simulink model "mmc"  (R2025a)
settings: Solver=VariableStepAuto  StartTime=0.0  StopTime=10  RelTol=1e-3
libraries: nesl_utility x145, ee_lib x103, fl_lib x100
(part 1 of 13)
settings Model: Creator=tanus  LastModifiedBy=tanus

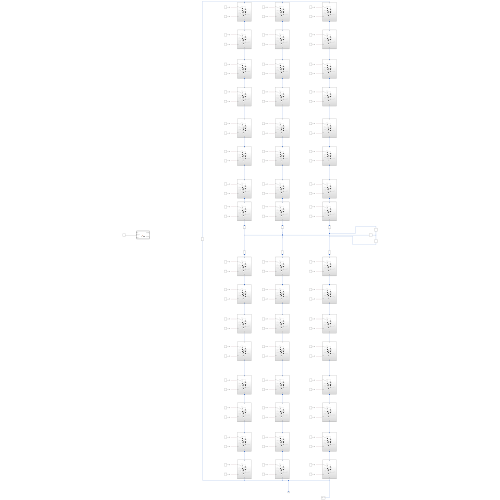
[thumbnail: Simulink's stored preview of the top-level diagram]
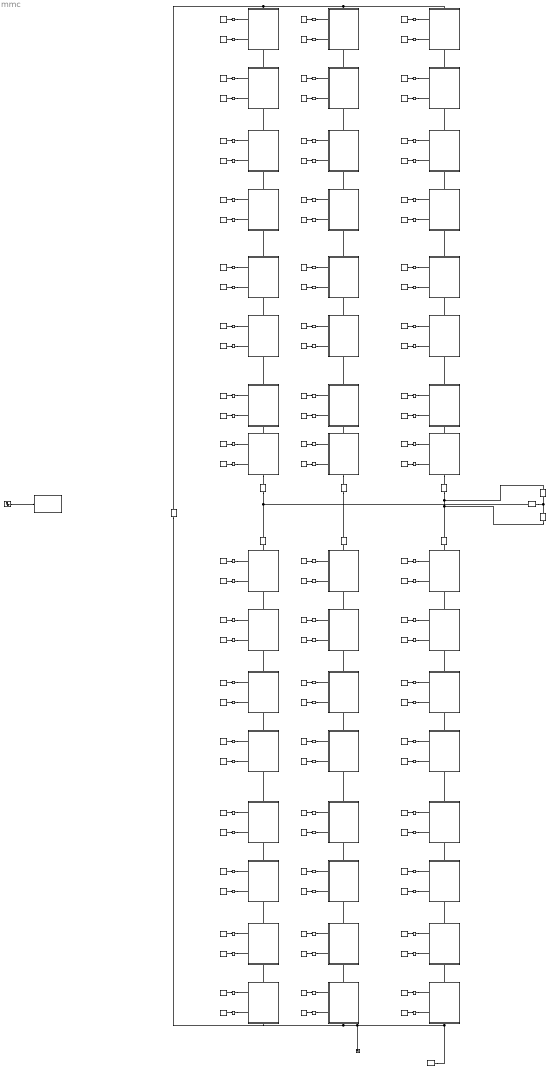
== system mmc ==
  Constant{1..96} (96 alike) : Constant  Value=10
  Electrical Reference : fl_lib/Electrical/Electrical Elements/Electrical Reference
  Inductor{6..11} (6 alike) : ee_lib/Passive/Inductor  l=1e-3 H  enable_L_tol=ee.enum.toleranceApplication.none  L_tol=20  tol_distribution=ee.enum.toleranceDistribution.uniform  nSigma=4  r=0 Ohm  g=1e-9 1/Ohm  enable_operating_limits=ee.enum.enable.no  operating_limit_action=ee.enum.passive.reportOpLim.warn  max_working_current=1 A  power_rating=1 W  i_L_specify=off  i_L_priority=High  i_L=0 A  i_L_nominal_specify=off  i_L_nominal_value=1  i_L_nominal_unit=A
  MATLAB Function : MATLAB Function  TreatAsAtomicUnit=on
  Resistor : fl_lib/Electrical/Electrical Elements/Resistor  R=1 Ohm  i_specify=off  i_priority=None  i=0 A  i_nominal_specify=off  i_nominal_value=1  i_nominal_unit=A  v_specify=off  v_priority=None  v=0 V  v_nominal_specify=off  v_nominal_value=1  v_nominal_unit=V
  Resistor1 : fl_lib/Electrical/Electrical Elements/Resistor  R=1 Ohm  i_specify=off  i_priority=None  i=0 A  i_nominal_specify=off  i_nominal_value=1  i_nominal_unit=A  v_specify=off  v_priority=None  v=0 V  v_nominal_specify=off  v_nominal_value=1  v_nominal_unit=V
  Resistor2 : fl_lib/Electrical/Electrical Elements/Resistor  R=1 Ohm  i_specify=off  i_priority=None  i=0 A  i_nominal_specify=off  i_nominal_value=1  i_nominal_unit=A  v_specify=off  v_priority=None  v=0 V  v_nominal_specify=off  v_nominal_value=1  v_nominal_unit=V
  Simulink-PS Converter{1..96} (96 alike) : nesl_utility/Simulink-PS Converter  PhysicalDomain=network_engine_domain  SubClassName=ps_input  LeftPortType=input  RightPortType=output  PseudoPeriodic=off  Frequencies=[]  NoiseDistribution=none  NoiseParameters=[]  Unit=1  AffineConversion=off  FilteringAndDerivatives=provide  SimscapeFilterOrder=1  InputFilterTimeConstant=0.001  UdotUserProvided=0
  Sine Wave : Sin  SampleTime=0
  Solver Configuration1 : nesl_utility/Solver Configuration  PhysicalDomain=network_engine_domain  SubClassName=solver  LeftPortType=input  RightPortType=generic  Tones=[]  Harmonics=[]  SimulateNoise=off  Profile=off  UseLocalSampling=off  EnableSwitchedLinearOptims=on  FrequencyDomain=off  UseCCode=off  RelTol=0.001  AbsTol=0.001  MinStep=1e-09  ToWorkspace=off  RevertToSquareIcSolve=off  NumHomotopyIterations=100  PhasorMode=off  PhasorModeNumHarmonics=1  ConsistencySolver=NEWTON_XTOL_AFTER_FTOL  IndexReductionMethod=DerivativeReplacement  DoDC=off  ResidualTolerance=1e-09  ConsistencyTolSource=GLOBAL  ConsistencyAbsTol=0.001  ConsistencyRelTol=0.001  ConsistencyTolFactor=0.001  UseLocalSolver=off  LocalSolverChoice=NE_BACKWARD_EULER_ADVANCER  ResolveIndetEquations=on  FunctionEvalNumThread=1  LocalSolverSampleTime=0.001  DoFixedCost=off  MaxNonlinIter=3  MaxModeIter=2  ComputeImpulses=off  ImpulseIterations=2  LinearAlgebra=auto  LinearAlgebraNumThread=0  EquationFormulation=NE_TIME_EF  DelaysMemoryBudget=1024  AutomaticFiltering=on  FilteringTimeConstant=0.001  PartitionStorageMethod=AS_NEEDED  PartitionMemoryBudget=1024  PartitionMethod=ROBUST  MultibodyUseLocalSolver=off  MultibodyLocalSolverChoice=ODE1  MultibodyLocalSolverSampleTime=0.001
  Subsystem1 : Subsystem
      settings: PortSchema="{\"entries\":[{\"content\":{\"sides\":[{\"content\":{\"connectorIds\":[\"LConn1\",\"LConn2\"]},\"type\":\"ConnectorPlacement.EquallySpacedRectSide\",\"uuid\":\"15b6a701-c482-4ab4-b894-e969b74b8fe7\"},{\"content\":{\"side\":\"RIGHT\"},\"type\":\"ConnectorPlacement.EquallySpacedRectSide\",\"uuid\":\"d0e695dd-06b6-4831-9b12-69abc92aa4b4\"},{\"content\":{\"connectorIds\":[\"LConn3\"],\"side\":\"TOP\"},\"type\":\"ConnectorPlacement.EquallySpacedRectSide\",\"uuid\":\"2d8cca64-5216-4108-8582-3d735b4d6af0\"},{\"content\":{\"connectorIds\":[\"RConn1\"],\"side\":\"BOTTOM\"},\"type\":\"ConnectorPlacement.EquallySpacedRectSide\",\"uuid\":\"da22ed5b-3a7b-44e1-acef-3ebda742cad5\"}]},\"type\":\"ConnectorPlacement.EquallySpacedConnector\",\"uuid\":\"49f96526-0040-486f-9e93-d2a8b3aa1224\"}],\"packageUris\":[\"http://schema.mathworks.com/mf0/Connector/R2020b\"],\"version\":\"1.0\"}"
  Subsystem10 : Subsystem
      settings: PortSchema="{\"entries\":[{\"content\":{\"sides\":[{\"content\":{\"connectorIds\":[\"LConn1\",\"LConn2\"]},\"type\":\"ConnectorPlacement.EquallySpacedRectSide\",\"uuid\":\"15b6a701-c482-4ab4-b894-e969b74b8fe7\"},{\"content\":{\"side\":\"RIGHT\"},\"type\":\"ConnectorPlacement.EquallySpacedRectSide\",\"uuid\":\"d0e695dd-06b6-4831-9b12-69abc92aa4b4\"},{\"content\":{\"connectorIds\":[\"LConn3\"],\"side\":\"TOP\"},\"type\":\"ConnectorPlacement.EquallySpacedRectSide\",\"uuid\":\"2d8cca64-5216-4108-8582-3d735b4d6af0\"},{\"content\":{\"connectorIds\":[\"RConn1\"],\"side\":\"BOTTOM\"},\"type\":\"ConnectorPlacement.EquallySpacedRectSide\",\"uuid\":\"da22ed5b-3a7b-44e1-acef-3ebda742cad5\"}]},\"type\":\"ConnectorPlacement.EquallySpacedConnector\",\"uuid\":\"49f96526-0040-486f-9e93-d2a8b3aa1224\"}],\"packageUris\":[\"http://schema.mathworks.com/mf0/Connector/R2020b\"],\"version\":\"1.0\"}"
  Subsystem11 : Subsystem
      settings: PortSchema="{\"entries\":[{\"content\":{\"sides\":[{\"content\":{\"connectorIds\":[\"LConn1\",\"LConn2\"]},\"type\":\"ConnectorPlacement.EquallySpacedRectSide\",\"uuid\":\"15b6a701-c482-4ab4-b894-e969b74b8fe7\"},{\"content\":{\"side\":\"RIGHT\"},\"type\":\"ConnectorPlacement.EquallySpacedRectSide\",\"uuid\":\"d0e695dd-06b6-4831-9b12-69abc92aa4b4\"},{\"content\":{\"connectorIds\":[\"LConn3\"],\"side\":\"TOP\"},\"type\":\"ConnectorPlacement.EquallySpacedRectSide\",\"uuid\":\"2d8cca64-5216-4108-8582-3d735b4d6af0\"},{\"content\":{\"connectorIds\":[\"RConn1\"],\"side\":\"BOTTOM\"},\"type\":\"ConnectorPlacement.EquallySpacedRectSide\",\"uuid\":\"da22ed5b-3a7b-44e1-acef-3ebda742cad5\"}]},\"type\":\"ConnectorPlacement.EquallySpacedConnector\",\"uuid\":\"49f96526-0040-486f-9e93-d2a8b3aa1224\"}],\"packageUris\":[\"http://schema.mathworks.com/mf0/Connector/R2020b\"],\"version\":\"1.0\"}"
  Subsystem12 : Subsystem
      settings: PortSchema="{\"entries\":[{\"content\":{\"sides\":[{\"content\":{\"connectorIds\":[\"LConn1\",\"LConn2\"]},\"type\":\"ConnectorPlacement.EquallySpacedRectSide\",\"uuid\":\"15b6a701-c482-4ab4-b894-e969b74b8fe7\"},{\"content\":{\"side\":\"RIGHT\"},\"type\":\"ConnectorPlacement.EquallySpacedRectSide\",\"uuid\":\"d0e695dd-06b6-4831-9b12-69abc92aa4b4\"},{\"content\":{\"connectorIds\":[\"LConn3\"],\"side\":\"TOP\"},\"type\":\"ConnectorPlacement.EquallySpacedRectSide\",\"uuid\":\"2d8cca64-5216-4108-8582-3d735b4d6af0\"},{\"content\":{\"connectorIds\":[\"RConn1\"],\"side\":\"BOTTOM\"},\"type\":\"ConnectorPlacement.EquallySpacedRectSide\",\"uuid\":\"da22ed5b-3a7b-44e1-acef-3ebda742cad5\"}]},\"type\":\"ConnectorPlacement.EquallySpacedConnector\",\"uuid\":\"49f96526-0040-486f-9e93-d2a8b3aa1224\"}],\"packageUris\":[\"http://schema.mathworks.com/mf0/Connector/R2020b\"],\"version\":\"1.0\"}"
  Subsystem13 : Subsystem
      settings: PortSchema="{\"entries\":[{\"content\":{\"sides\":[{\"content\":{\"connectorIds\":[\"LConn1\",\"LConn2\"]},\"type\":\"ConnectorPlacement.EquallySpacedRectSide\",\"uuid\":\"15b6a701-c482-4ab4-b894-e969b74b8fe7\"},{\"content\":{\"side\":\"RIGHT\"},\"type\":\"ConnectorPlacement.EquallySpacedRectSide\",\"uuid\":\"d0e695dd-06b6-4831-9b12-69abc92aa4b4\"},{\"content\":{\"connectorIds\":[\"LConn3\"],\"side\":\"TOP\"},\"type\":\"ConnectorPlacement.EquallySpacedRectSide\",\"uuid\":\"2d8cca64-5216-4108-8582-3d735b4d6af0\"},{\"content\":{\"connectorIds\":[\"RConn1\"],\"side\":\"BOTTOM\"},\"type\":\"ConnectorPlacement.EquallySpacedRectSide\",\"uuid\":\"da22ed5b-3a7b-44e1-acef-3ebda742cad5\"}]},\"type\":\"ConnectorPlacement.EquallySpacedConnector\",\"uuid\":\"49f96526-0040-486f-9e93-d2a8b3aa1224\"}],\"packageUris\":[\"http://schema.mathworks.com/mf0/Connector/R2020b\"],\"version\":\"1.0\"}"
  Subsystem14 : Subsystem
      settings: PortSchema="{\"entries\":[{\"content\":{\"sides\":[{\"content\":{\"connectorIds\":[\"LConn1\",\"LConn2\"]},\"type\":\"ConnectorPlacement.EquallySpacedRectSide\",\"uuid\":\"15b6a701-c482-4ab4-b894-e969b74b8fe7\"},{\"content\":{\"side\":\"RIGHT\"},\"type\":\"ConnectorPlacement.EquallySpacedRectSide\",\"uuid\":\"d0e695dd-06b6-4831-9b12-69abc92aa4b4\"},{\"content\":{\"connectorIds\":[\"LConn3\"],\"side\":\"TOP\"},\"type\":\"ConnectorPlacement.EquallySpacedRectSide\",\"uuid\":\"2d8cca64-5216-4108-8582-3d735b4d6af0\"},{\"content\":{\"connectorIds\":[\"RConn1\"],\"side\":\"BOTTOM\"},\"type\":\"ConnectorPlacement.EquallySpacedRectSide\",\"uuid\":\"da22ed5b-3a7b-44e1-acef-3ebda742cad5\"}]},\"type\":\"ConnectorPlacement.EquallySpacedConnector\",\"uuid\":\"49f96526-0040-486f-9e93-d2a8b3aa1224\"}],\"packageUris\":[\"http://schema.mathworks.com/mf0/Connector/R2020b\"],\"version\":\"1.0\"}"
  Subsystem15 : Subsystem
      settings: PortSchema="{\"entries\":[{\"content\":{\"sides\":[{\"content\":{\"connectorIds\":[\"LConn1\",\"LConn2\"]},\"type\":\"ConnectorPlacement.EquallySpacedRectSide\",\"uuid\":\"15b6a701-c482-4ab4-b894-e969b74b8fe7\"},{\"content\":{\"side\":\"RIGHT\"},\"type\":\"ConnectorPlacement.EquallySpacedRectSide\",\"uuid\":\"d0e695dd-06b6-4831-9b12-69abc92aa4b4\"},{\"content\":{\"connectorIds\":[\"LConn3\"],\"side\":\"TOP\"},\"type\":\"ConnectorPlacement.EquallySpacedRectSide\",\"uuid\":\"2d8cca64-5216-4108-8582-3d735b4d6af0\"},{\"content\":{\"connectorIds\":[\"RConn1\"],\"side\":\"BOTTOM\"},\"type\":\"ConnectorPlacement.EquallySpacedRectSide\",\"uuid\":\"da22ed5b-3a7b-44e1-acef-3ebda742cad5\"}]},\"type\":\"ConnectorPlacement.EquallySpacedConnector\",\"uuid\":\"49f96526-0040-486f-9e93-d2a8b3aa1224\"}],\"packageUris\":[\"http://schema.mathworks.com/mf0/Connector/R2020b\"],\"version\":\"1.0\"}"
  Subsystem16 : Subsystem
      settings: PortSchema="{\"entries\":[{\"content\":{\"sides\":[{\"content\":{\"connectorIds\":[\"LConn1\",\"LConn2\"]},\"type\":\"ConnectorPlacement.EquallySpacedRectSide\",\"uuid\":\"15b6a701-c482-4ab4-b894-e969b74b8fe7\"},{\"content\":{\"side\":\"RIGHT\"},\"type\":\"ConnectorPlacement.EquallySpacedRectSide\",\"uuid\":\"d0e695dd-06b6-4831-9b12-69abc92aa4b4\"},{\"content\":{\"connectorIds\":[\"LConn3\"],\"side\":\"TOP\"},\"type\":\"ConnectorPlacement.EquallySpacedRectSide\",\"uuid\":\"2d8cca64-5216-4108-8582-3d735b4d6af0\"},{\"content\":{\"connectorIds\":[\"RConn1\"],\"side\":\"BOTTOM\"},\"type\":\"ConnectorPlacement.EquallySpacedRectSide\",\"uuid\":\"da22ed5b-3a7b-44e1-acef-3ebda742cad5\"}]},\"type\":\"ConnectorPlacement.EquallySpacedConnector\",\"uuid\":\"49f96526-0040-486f-9e93-d2a8b3aa1224\"}],\"packageUris\":[\"http://schema.mathworks.com/mf0/Connector/R2020b\"],\"version\":\"1.0\"}"
  Subsystem17 : Subsystem
      settings: PortSchema="{\"entries\":[{\"content\":{\"sides\":[{\"content\":{\"connectorIds\":[\"LConn1\",\"LConn2\"]},\"type\":\"ConnectorPlacement.EquallySpacedRectSide\",\"uuid\":\"15b6a701-c482-4ab4-b894-e969b74b8fe7\"},{\"content\":{\"side\":\"RIGHT\"},\"type\":\"ConnectorPlacement.EquallySpacedRectSide\",\"uuid\":\"d0e695dd-06b6-4831-9b12-69abc92aa4b4\"},{\"content\":{\"connectorIds\":[\"LConn3\"],\"side\":\"TOP\"},\"type\":\"ConnectorPlacement.EquallySpacedRectSide\",\"uuid\":\"2d8cca64-5216-4108-8582-3d735b4d6af0\"},{\"content\":{\"connectorIds\":[\"RConn1\"],\"side\":\"BOTTOM\"},\"type\":\"ConnectorPlacement.EquallySpacedRectSide\",\"uuid\":\"da22ed5b-3a7b-44e1-acef-3ebda742cad5\"}]},\"type\":\"ConnectorPlacement.EquallySpacedConnector\",\"uuid\":\"49f96526-0040-486f-9e93-d2a8b3aa1224\"}],\"packageUris\":[\"http://schema.mathworks.com/mf0/Connector/R2020b\"],\"version\":\"1.0\"}"
  Subsystem18 : Subsystem
      settings: PortSchema="{\"entries\":[{\"content\":{\"sides\":[{\"content\":{\"connectorIds\":[\"LConn1\",\"LConn2\"]},\"type\":\"ConnectorPlacement.EquallySpacedRectSide\",\"uuid\":\"15b6a701-c482-4ab4-b894-e969b74b8fe7\"},{\"content\":{\"side\":\"RIGHT\"},\"type\":\"ConnectorPlacement.EquallySpacedRectSide\",\"uuid\":\"d0e695dd-06b6-4831-9b12-69abc92aa4b4\"},{\"content\":{\"connectorIds\":[\"LConn3\"],\"side\":\"TOP\"},\"type\":\"ConnectorPlacement.EquallySpacedRectSide\",\"uuid\":\"2d8cca64-5216-4108-8582-3d735b4d6af0\"},{\"content\":{\"connectorIds\":[\"RConn1\"],\"side\":\"BOTTOM\"},\"type\":\"ConnectorPlacement.EquallySpacedRectSide\",\"uuid\":\"da22ed5b-3a7b-44e1-acef-3ebda742cad5\"}]},\"type\":\"ConnectorPlacement.EquallySpacedConnector\",\"uuid\":\"49f96526-0040-486f-9e93-d2a8b3aa1224\"}],\"packageUris\":[\"http://schema.mathworks.com/mf0/Connector/R2020b\"],\"version\":\"1.0\"}"
  Subsystem19 : Subsystem
      settings: PortSchema="{\"entries\":[{\"content\":{\"sides\":[{\"content\":{\"connectorIds\":[\"LConn1\",\"LConn2\"]},\"type\":\"ConnectorPlacement.EquallySpacedRectSide\",\"uuid\":\"15b6a701-c482-4ab4-b894-e969b74b8fe7\"},{\"content\":{\"side\":\"RIGHT\"},\"type\":\"ConnectorPlacement.EquallySpacedRectSide\",\"uuid\":\"d0e695dd-06b6-4831-9b12-69abc92aa4b4\"},{\"content\":{\"connectorIds\":[\"LConn3\"],\"side\":\"TOP\"},\"type\":\"ConnectorPlacement.EquallySpacedRectSide\",\"uuid\":\"2d8cca64-5216-4108-8582-3d735b4d6af0\"},{\"content\":{\"connectorIds\":[\"RConn1\"],\"side\":\"BOTTOM\"},\"type\":\"ConnectorPlacement.EquallySpacedRectSide\",\"uuid\":\"da22ed5b-3a7b-44e1-acef-3ebda742cad5\"}]},\"type\":\"ConnectorPlacement.EquallySpacedConnector\",\"uuid\":\"49f96526-0040-486f-9e93-d2a8b3aa1224\"}],\"packageUris\":[\"http://schema.mathworks.com/mf0/Connector/R2020b\"],\"version\":\"1.0\"}"
  Subsystem2 : Subsystem
      settings: PortSchema="{\"entries\":[{\"content\":{\"sides\":[{\"content\":{\"connectorIds\":[\"LConn1\",\"LConn2\"]},\"type\":\"ConnectorPlacement.EquallySpacedRectSide\",\"uuid\":\"15b6a701-c482-4ab4-b894-e969b74b8fe7\"},{\"content\":{\"side\":\"RIGHT\"},\"type\":\"ConnectorPlacement.EquallySpacedRectSide\",\"uuid\":\"d0e695dd-06b6-4831-9b12-69abc92aa4b4\"},{\"content\":{\"connectorIds\":[\"LConn3\"],\"side\":\"TOP\"},\"type\":\"ConnectorPlacement.EquallySpacedRectSide\",\"uuid\":\"2d8cca64-5216-4108-8582-3d735b4d6af0\"},{\"content\":{\"connectorIds\":[\"RConn1\"],\"side\":\"BOTTOM\"},\"type\":\"ConnectorPlacement.EquallySpacedRectSide\",\"uuid\":\"da22ed5b-3a7b-44e1-acef-3ebda742cad5\"}]},\"type\":\"ConnectorPlacement.EquallySpacedConnector\",\"uuid\":\"49f96526-0040-486f-9e93-d2a8b3aa1224\"}],\"packageUris\":[\"http://schema.mathworks.com/mf0/Connector/R2020b\"],\"version\":\"1.0\"}"
  Subsystem20 : Subsystem
      settings: PortSchema="{\"entries\":[{\"content\":{\"sides\":[{\"content\":{\"connectorIds\":[\"LConn1\",\"LConn2\"]},\"type\":\"ConnectorPlacement.EquallySpacedRectSide\",\"uuid\":\"15b6a701-c482-4ab4-b894-e969b74b8fe7\"},{\"content\":{\"side\":\"RIGHT\"},\"type\":\"ConnectorPlacement.EquallySpacedRectSide\",\"uuid\":\"d0e695dd-06b6-4831-9b12-69abc92aa4b4\"},{\"content\":{\"connectorIds\":[\"LConn3\"],\"side\":\"TOP\"},\"type\":\"ConnectorPlacement.EquallySpacedRectSide\",\"uuid\":\"2d8cca64-5216-4108-8582-3d735b4d6af0\"},{\"content\":{\"connectorIds\":[\"RConn1\"],\"side\":\"BOTTOM\"},\"type\":\"ConnectorPlacement.EquallySpacedRectSide\",\"uuid\":\"da22ed5b-3a7b-44e1-acef-3ebda742cad5\"}]},\"type\":\"ConnectorPlacement.EquallySpacedConnector\",\"uuid\":\"49f96526-0040-486f-9e93-d2a8b3aa1224\"}],\"packageUris\":[\"http://schema.mathworks.com/mf0/Connector/R2020b\"],\"version\":\"1.0\"}"
  Subsystem21 : Subsystem
      settings: PortSchema="{\"entries\":[{\"content\":{\"sides\":[{\"content\":{\"connectorIds\":[\"LConn1\",\"LConn2\"]},\"type\":\"ConnectorPlacement.EquallySpacedRectSide\",\"uuid\":\"15b6a701-c482-4ab4-b894-e969b74b8fe7\"},{\"content\":{\"side\":\"RIGHT\"},\"type\":\"ConnectorPlacement.EquallySpacedRectSide\",\"uuid\":\"d0e695dd-06b6-4831-9b12-69abc92aa4b4\"},{\"content\":{\"connectorIds\":[\"LConn3\"],\"side\":\"TOP\"},\"type\":\"ConnectorPlacement.EquallySpacedRectSide\",\"uuid\":\"2d8cca64-5216-4108-8582-3d735b4d6af0\"},{\"content\":{\"connectorIds\":[\"RConn1\"],\"side\":\"BOTTOM\"},\"type\":\"ConnectorPlacement.EquallySpacedRectSide\",\"uuid\":\"da22ed5b-3a7b-44e1-acef-3ebda742cad5\"}]},\"type\":\"ConnectorPlacement.EquallySpacedConnector\",\"uuid\":\"49f96526-0040-486f-9e93-d2a8b3aa1224\"}],\"packageUris\":[\"http://schema.mathworks.com/mf0/Connector/R2020b\"],\"version\":\"1.0\"}"
  Subsystem22 : Subsystem
      settings: PortSchema="{\"entries\":[{\"content\":{\"sides\":[{\"content\":{\"connectorIds\":[\"LConn1\",\"LConn2\"]},\"type\":\"ConnectorPlacement.EquallySpacedRectSide\",\"uuid\":\"15b6a701-c482-4ab4-b894-e969b74b8fe7\"},{\"content\":{\"side\":\"RIGHT\"},\"type\":\"ConnectorPlacement.EquallySpacedRectSide\",\"uuid\":\"d0e695dd-06b6-4831-9b12-69abc92aa4b4\"},{\"content\":{\"connectorIds\":[\"LConn3\"],\"side\":\"TOP\"},\"type\":\"ConnectorPlacement.EquallySpacedRectSide\",\"uuid\":\"2d8cca64-5216-4108-8582-3d735b4d6af0\"},{\"content\":{\"connectorIds\":[\"RConn1\"],\"side\":\"BOTTOM\"},\"type\":\"ConnectorPlacement.EquallySpacedRectSide\",\"uuid\":\"da22ed5b-3a7b-44e1-acef-3ebda742cad5\"}]},\"type\":\"ConnectorPlacement.EquallySpacedConnector\",\"uuid\":\"49f96526-0040-486f-9e93-d2a8b3aa1224\"}],\"packageUris\":[\"http://schema.mathworks.com/mf0/Connector/R2020b\"],\"version\":\"1.0\"}"
  Subsystem23 : Subsystem
      settings: PortSchema="{\"entries\":[{\"content\":{\"sides\":[{\"content\":{\"connectorIds\":[\"LConn1\",\"LConn2\"]},\"type\":\"ConnectorPlacement.EquallySpacedRectSide\",\"uuid\":\"15b6a701-c482-4ab4-b894-e969b74b8fe7\"},{\"content\":{\"side\":\"RIGHT\"},\"type\":\"ConnectorPlacement.EquallySpacedRectSide\",\"uuid\":\"d0e695dd-06b6-4831-9b12-69abc92aa4b4\"},{\"content\":{\"connectorIds\":[\"LConn3\"],\"side\":\"TOP\"},\"type\":\"ConnectorPlacement.EquallySpacedRectSide\",\"uuid\":\"2d8cca64-5216-4108-8582-3d735b4d6af0\"},{\"content\":{\"connectorIds\":[\"RConn1\"],\"side\":\"BOTTOM\"},\"type\":\"ConnectorPlacement.EquallySpacedRectSide\",\"uuid\":\"da22ed5b-3a7b-44e1-acef-3ebda742cad5\"}]},\"type\":\"ConnectorPlacement.EquallySpacedConnector\",\"uuid\":\"49f96526-0040-486f-9e93-d2a8b3aa1224\"}],\"packageUris\":[\"http://schema.mathworks.com/mf0/Connector/R2020b\"],\"version\":\"1.0\"}"
  Subsystem24 : Subsystem
      settings: PortSchema="{\"entries\":[{\"content\":{\"sides\":[{\"content\":{\"connectorIds\":[\"LConn1\",\"LConn2\"]},\"type\":\"ConnectorPlacement.EquallySpacedRectSide\",\"uuid\":\"15b6a701-c482-4ab4-b894-e969b74b8fe7\"},{\"content\":{\"side\":\"RIGHT\"},\"type\":\"ConnectorPlacement.EquallySpacedRectSide\",\"uuid\":\"d0e695dd-06b6-4831-9b12-69abc92aa4b4\"},{\"content\":{\"connectorIds\":[\"LConn3\"],\"side\":\"TOP\"},\"type\":\"ConnectorPlacement.EquallySpacedRectSide\",\"uuid\":\"2d8cca64-5216-4108-8582-3d735b4d6af0\"},{\"content\":{\"connectorIds\":[\"RConn1\"],\"side\":\"BOTTOM\"},\"type\":\"ConnectorPlacement.EquallySpacedRectSide\",\"uuid\":\"da22ed5b-3a7b-44e1-acef-3ebda742cad5\"}]},\"type\":\"ConnectorPlacement.EquallySpacedConnector\",\"uuid\":\"49f96526-0040-486f-9e93-d2a8b3aa1224\"}],\"packageUris\":[\"http://schema.mathworks.com/mf0/Connector/R2020b\"],\"version\":\"1.0\"}"
  Subsystem25 : Subsystem
      settings: PortSchema="{\"entries\":[{\"content\":{\"sides\":[{\"content\":{\"connectorIds\":[\"LConn1\",\"LConn2\"]},\"type\":\"ConnectorPlacement.EquallySpacedRectSide\",\"uuid\":\"15b6a701-c482-4ab4-b894-e969b74b8fe7\"},{\"content\":{\"side\":\"RIGHT\"},\"type\":\"ConnectorPlacement.EquallySpacedRectSide\",\"uuid\":\"d0e695dd-06b6-4831-9b12-69abc92aa4b4\"},{\"content\":{\"connectorIds\":[\"LConn3\"],\"side\":\"TOP\"},\"type\":\"ConnectorPlacement.EquallySpacedRectSide\",\"uuid\":\"2d8cca64-5216-4108-8582-3d735b4d6af0\"},{\"content\":{\"connectorIds\":[\"RConn1\"],\"side\":\"BOTTOM\"},\"type\":\"ConnectorPlacement.EquallySpacedRectSide\",\"uuid\":\"da22ed5b-3a7b-44e1-acef-3ebda742cad5\"}]},\"type\":\"ConnectorPlacement.EquallySpacedConnector\",\"uuid\":\"49f96526-0040-486f-9e93-d2a8b3aa1224\"}],\"packageUris\":[\"http://schema.mathworks.com/mf0/Connector/R2020b\"],\"version\":\"1.0\"}"
  Subsystem26 : Subsystem
      settings: PortSchema="{\"entries\":[{\"content\":{\"sides\":[{\"content\":{\"connectorIds\":[\"LConn1\",\"LConn2\"]},\"type\":\"ConnectorPlacement.EquallySpacedRectSide\",\"uuid\":\"15b6a701-c482-4ab4-b894-e969b74b8fe7\"},{\"content\":{\"side\":\"RIGHT\"},\"type\":\"ConnectorPlacement.EquallySpacedRectSide\",\"uuid\":\"d0e695dd-06b6-4831-9b12-69abc92aa4b4\"},{\"content\":{\"connectorIds\":[\"LConn3\"],\"side\":\"TOP\"},\"type\":\"ConnectorPlacement.EquallySpacedRectSide\",\"uuid\":\"2d8cca64-5216-4108-8582-3d735b4d6af0\"},{\"content\":{\"connectorIds\":[\"RConn1\"],\"side\":\"BOTTOM\"},\"type\":\"ConnectorPlacement.EquallySpacedRectSide\",\"uuid\":\"da22ed5b-3a7b-44e1-acef-3ebda742cad5\"}]},\"type\":\"ConnectorPlacement.EquallySpacedConnector\",\"uuid\":\"49f96526-0040-486f-9e93-d2a8b3aa1224\"}],\"packageUris\":[\"http://schema.mathworks.com/mf0/Connector/R2020b\"],\"version\":\"1.0\"}"
  Subsystem27 : Subsystem
      settings: PortSchema="{\"entries\":[{\"content\":{\"sides\":[{\"content\":{\"connectorIds\":[\"LConn1\",\"LConn2\"]},\"type\":\"ConnectorPlacement.EquallySpacedRectSide\",\"uuid\":\"15b6a701-c482-4ab4-b894-e969b74b8fe7\"},{\"content\":{\"side\":\"RIGHT\"},\"type\":\"ConnectorPlacement.EquallySpacedRectSide\",\"uuid\":\"d0e695dd-06b6-4831-9b12-69abc92aa4b4\"},{\"content\":{\"connectorIds\":[\"LConn3\"],\"side\":\"TOP\"},\"type\":\"ConnectorPlacement.EquallySpacedRectSide\",\"uuid\":\"2d8cca64-5216-4108-8582-3d735b4d6af0\"},{\"content\":{\"connectorIds\":[\"RConn1\"],\"side\":\"BOTTOM\"},\"type\":\"ConnectorPlacement.EquallySpacedRectSide\",\"uuid\":\"da22ed5b-3a7b-44e1-acef-3ebda742cad5\"}]},\"type\":\"ConnectorPlacement.EquallySpacedConnector\",\"uuid\":\"49f96526-0040-486f-9e93-d2a8b3aa1224\"}],\"packageUris\":[\"http://schema.mathworks.com/mf0/Connector/R2020b\"],\"version\":\"1.0\"}"
  Subsystem28 : Subsystem
      settings: PortSchema="{\"entries\":[{\"content\":{\"sides\":[{\"content\":{\"connectorIds\":[\"LConn1\",\"LConn2\"]},\"type\":\"ConnectorPlacement.EquallySpacedRectSide\",\"uuid\":\"15b6a701-c482-4ab4-b894-e969b74b8fe7\"},{\"content\":{\"side\":\"RIGHT\"},\"type\":\"ConnectorPlacement.EquallySpacedRectSide\",\"uuid\":\"d0e695dd-06b6-4831-9b12-69abc92aa4b4\"},{\"content\":{\"connectorIds\":[\"LConn3\"],\"side\":\"TOP\"},\"type\":\"ConnectorPlacement.EquallySpacedRectSide\",\"uuid\":\"2d8cca64-5216-4108-8582-3d735b4d6af0\"},{\"content\":{\"connectorIds\":[\"RConn1\"],\"side\":\"BOTTOM\"},\"type\":\"ConnectorPlacement.EquallySpacedRectSide\",\"uuid\":\"da22ed5b-3a7b-44e1-acef-3ebda742cad5\"}]},\"type\":\"ConnectorPlacement.EquallySpacedConnector\",\"uuid\":\"49f96526-0040-486f-9e93-d2a8b3aa1224\"}],\"packageUris\":[\"http://schema.mathworks.com/mf0/Connector/R2020b\"],\"version\":\"1.0\"}"
  Subsystem29 : Subsystem
      settings: PortSchema="{\"entries\":[{\"content\":{\"sides\":[{\"content\":{\"connectorIds\":[\"LConn1\",\"LConn2\"]},\"type\":\"ConnectorPlacement.EquallySpacedRectSide\",\"uuid\":\"15b6a701-c482-4ab4-b894-e969b74b8fe7\"},{\"content\":{\"side\":\"RIGHT\"},\"type\":\"ConnectorPlacement.EquallySpacedRectSide\",\"uuid\":\"d0e695dd-06b6-4831-9b12-69abc92aa4b4\"},{\"content\":{\"connectorIds\":[\"LConn3\"],\"side\":\"TOP\"},\"type\":\"ConnectorPlacement.EquallySpacedRectSide\",\"uuid\":\"2d8cca64-5216-4108-8582-3d735b4d6af0\"},{\"content\":{\"connectorIds\":[\"RConn1\"],\"side\":\"BOTTOM\"},\"type\":\"ConnectorPlacement.EquallySpacedRectSide\",\"uuid\":\"da22ed5b-3a7b-44e1-acef-3ebda742cad5\"}]},\"type\":\"ConnectorPlacement.EquallySpacedConnector\",\"uuid\":\"49f96526-0040-486f-9e93-d2a8b3aa1224\"}],\"packageUris\":[\"http://schema.mathworks.com/mf0/Connector/R2020b\"],\"version\":\"1.0\"}"
  Subsystem3 : Subsystem
      settings: PortSchema="{\"entries\":[{\"content\":{\"sides\":[{\"content\":{\"connectorIds\":[\"LConn1\",\"LConn2\"]},\"type\":\"ConnectorPlacement.EquallySpacedRectSide\",\"uuid\":\"15b6a701-c482-4ab4-b894-e969b74b8fe7\"},{\"content\":{\"side\":\"RIGHT\"},\"type\":\"ConnectorPlacement.EquallySpacedRectSide\",\"uuid\":\"d0e695dd-06b6-4831-9b12-69abc92aa4b4\"},{\"content\":{\"connectorIds\":[\"LConn3\"],\"side\":\"TOP\"},\"type\":\"ConnectorPlacement.EquallySpacedRectSide\",\"uuid\":\"2d8cca64-5216-4108-8582-3d735b4d6af0\"},{\"content\":{\"connectorIds\":[\"RConn1\"],\"side\":\"BOTTOM\"},\"type\":\"ConnectorPlacement.EquallySpacedRectSide\",\"uuid\":\"da22ed5b-3a7b-44e1-acef-3ebda742cad5\"}]},\"type\":\"ConnectorPlacement.EquallySpacedConnector\",\"uuid\":\"49f96526-0040-486f-9e93-d2a8b3aa1224\"}],\"packageUris\":[\"http://schema.mathworks.com/mf0/Connector/R2020b\"],\"version\":\"1.0\"}"
  Subsystem30 : Subsystem
      settings: PortSchema="{\"entries\":[{\"content\":{\"sides\":[{\"content\":{\"connectorIds\":[\"LConn1\",\"LConn2\"]},\"type\":\"ConnectorPlacement.EquallySpacedRectSide\",\"uuid\":\"15b6a701-c482-4ab4-b894-e969b74b8fe7\"},{\"content\":{\"side\":\"RIGHT\"},\"type\":\"ConnectorPlacement.EquallySpacedRectSide\",\"uuid\":\"d0e695dd-06b6-4831-9b12-69abc92aa4b4\"},{\"content\":{\"connectorIds\":[\"LConn3\"],\"side\":\"TOP\"},\"type\":\"ConnectorPlacement.EquallySpacedRectSide\",\"uuid\":\"2d8cca64-5216-4108-8582-3d735b4d6af0\"},{\"content\":{\"connectorIds\":[\"RConn1\"],\"side\":\"BOTTOM\"},\"type\":\"ConnectorPlacement.EquallySpacedRectSide\",\"uuid\":\"da22ed5b-3a7b-44e1-acef-3ebda742cad5\"}]},\"type\":\"ConnectorPlacement.EquallySpacedConnector\",\"uuid\":\"49f96526-0040-486f-9e93-d2a8b3aa1224\"}],\"packageUris\":[\"http://schema.mathworks.com/mf0/Connector/R2020b\"],\"version\":\"1.0\"}"
  Subsystem31 : Subsystem
      settings: PortSchema="{\"entries\":[{\"content\":{\"sides\":[{\"content\":{\"connectorIds\":[\"LConn1\",\"LConn2\"]},\"type\":\"ConnectorPlacement.EquallySpacedRectSide\",\"uuid\":\"15b6a701-c482-4ab4-b894-e969b74b8fe7\"},{\"content\":{\"side\":\"RIGHT\"},\"type\":\"ConnectorPlacement.EquallySpacedRectSide\",\"uuid\":\"d0e695dd-06b6-4831-9b12-69abc92aa4b4\"},{\"content\":{\"connectorIds\":[\"LConn3\"],\"side\":\"TOP\"},\"type\":\"ConnectorPlacement.EquallySpacedRectSide\",\"uuid\":\"2d8cca64-5216-4108-8582-3d735b4d6af0\"},{\"content\":{\"connectorIds\":[\"RConn1\"],\"side\":\"BOTTOM\"},\"type\":\"ConnectorPlacement.EquallySpacedRectSide\",\"uuid\":\"da22ed5b-3a7b-44e1-acef-3ebda742cad5\"}]},\"type\":\"ConnectorPlacement.EquallySpacedConnector\",\"uuid\":\"49f96526-0040-486f-9e93-d2a8b3aa1224\"}],\"packageUris\":[\"http://schema.mathworks.com/mf0/Connector/R2020b\"],\"version\":\"1.0\"}"
  Subsystem32 : Subsystem
      settings: PortSchema="{\"entries\":[{\"content\":{\"sides\":[{\"content\":{\"connectorIds\":[\"LConn1\",\"LConn2\"]},\"type\":\"ConnectorPlacement.EquallySpacedRectSide\",\"uuid\":\"15b6a701-c482-4ab4-b894-e969b74b8fe7\"},{\"content\":{\"side\":\"RIGHT\"},\"type\":\"ConnectorPlacement.EquallySpacedRectSide\",\"uuid\":\"d0e695dd-06b6-4831-9b12-69abc92aa4b4\"},{\"content\":{\"connectorIds\":[\"LConn3\"],\"side\":\"TOP\"},\"type\":\"ConnectorPlacement.EquallySpacedRectSide\",\"uuid\":\"2d8cca64-5216-4108-8582-3d735b4d6af0\"},{\"content\":{\"connectorIds\":[\"RConn1\"],\"side\":\"BOTTOM\"},\"type\":\"ConnectorPlacement.EquallySpacedRectSide\",\"uuid\":\"da22ed5b-3a7b-44e1-acef-3ebda742cad5\"}]},\"type\":\"ConnectorPlacement.EquallySpacedConnector\",\"uuid\":\"49f96526-0040-486f-9e93-d2a8b3aa1224\"}],\"packageUris\":[\"http://schema.mathworks.com/mf0/Connector/R2020b\"],\"version\":\"1.0\"}"
  Subsystem33 : Subsystem
      settings: PortSchema="{\"entries\":[{\"content\":{\"sides\":[{\"content\":{\"connectorIds\":[\"LConn1\",\"LConn2\"]},\"type\":\"ConnectorPlacement.EquallySpacedRectSide\",\"uuid\":\"15b6a701-c482-4ab4-b894-e969b74b8fe7\"},{\"content\":{\"side\":\"RIGHT\"},\"type\":\"ConnectorPlacement.EquallySpacedRectSide\",\"uuid\":\"d0e695dd-06b6-4831-9b12-69abc92aa4b4\"},{\"content\":{\"connectorIds\":[\"LConn3\"],\"side\":\"TOP\"},\"type\":\"ConnectorPlacement.EquallySpacedRectSide\",\"uuid\":\"2d8cca64-5216-4108-8582-3d735b4d6af0\"},{\"content\":{\"connectorIds\":[\"RConn1\"],\"side\":\"BOTTOM\"},\"type\":\"ConnectorPlacement.EquallySpacedRectSide\",\"uuid\":\"da22ed5b-3a7b-44e1-acef-3ebda742cad5\"}]},\"type\":\"ConnectorPlacement.EquallySpacedConnector\",\"uuid\":\"49f96526-0040-486f-9e93-d2a8b3aa1224\"}],\"packageUris\":[\"http://schema.mathworks.com/mf0/Connector/R2020b\"],\"version\":\"1.0\"}"
  Subsystem34 : Subsystem
      settings: PortSchema="{\"entries\":[{\"content\":{\"sides\":[{\"content\":{\"connectorIds\":[\"LConn1\",\"LConn2\"]},\"type\":\"ConnectorPlacement.EquallySpacedRectSide\",\"uuid\":\"15b6a701-c482-4ab4-b894-e969b74b8fe7\"},{\"content\":{\"side\":\"RIGHT\"},\"type\":\"ConnectorPlacement.EquallySpacedRectSide\",\"uuid\":\"d0e695dd-06b6-4831-9b12-69abc92aa4b4\"},{\"content\":{\"connectorIds\":[\"LConn3\"],\"side\":\"TOP\"},\"type\":\"ConnectorPlacement.EquallySpacedRectSide\",\"uuid\":\"2d8cca64-5216-4108-8582-3d735b4d6af0\"},{\"content\":{\"connectorIds\":[\"RConn1\"],\"side\":\"BOTTOM\"},\"type\":\"ConnectorPlacement.EquallySpacedRectSide\",\"uuid\":\"da22ed5b-3a7b-44e1-acef-3ebda742cad5\"}]},\"type\":\"ConnectorPlacement.EquallySpacedConnector\",\"uuid\":\"49f96526-0040-486f-9e93-d2a8b3aa1224\"}],\"packageUris\":[\"http://schema.mathworks.com/mf0/Connector/R2020b\"],\"version\":\"1.0\"}"
  Subsystem35 : Subsystem
      settings: PortSchema="{\"entries\":[{\"content\":{\"sides\":[{\"content\":{\"connectorIds\":[\"LConn1\",\"LConn2\"]},\"type\":\"ConnectorPlacement.EquallySpacedRectSide\",\"uuid\":\"15b6a701-c482-4ab4-b894-e969b74b8fe7\"},{\"content\":{\"side\":\"RIGHT\"},\"type\":\"ConnectorPlacement.EquallySpacedRectSide\",\"uuid\":\"d0e695dd-06b6-4831-9b12-69abc92aa4b4\"},{\"content\":{\"connectorIds\":[\"LConn3\"],\"side\":\"TOP\"},\"type\":\"ConnectorPlacement.EquallySpacedRectSide\",\"uuid\":\"2d8cca64-5216-4108-8582-3d735b4d6af0\"},{\"content\":{\"connectorIds\":[\"RConn1\"],\"side\":\"BOTTOM\"},\"type\":\"ConnectorPlacement.EquallySpacedRectSide\",\"uuid\":\"da22ed5b-3a7b-44e1-acef-3ebda742cad5\"}]},\"type\":\"ConnectorPlacement.EquallySpacedConnector\",\"uuid\":\"49f96526-0040-486f-9e93-d2a8b3aa1224\"}],\"packageUris\":[\"http://schema.mathworks.com/mf0/Connector/R2020b\"],\"version\":\"1.0\"}"
  Subsystem36 : Subsystem
      settings: PortSchema="{\"entries\":[{\"content\":{\"sides\":[{\"content\":{\"connectorIds\":[\"LConn1\",\"LConn2\"]},\"type\":\"ConnectorPlacement.EquallySpacedRectSide\",\"uuid\":\"15b6a701-c482-4ab4-b894-e969b74b8fe7\"},{\"content\":{\"side\":\"RIGHT\"},\"type\":\"ConnectorPlacement.EquallySpacedRectSide\",\"uuid\":\"d0e695dd-06b6-4831-9b12-69abc92aa4b4\"},{\"content\":{\"connectorIds\":[\"LConn3\"],\"side\":\"TOP\"},\"type\":\"ConnectorPlacement.EquallySpacedRectSide\",\"uuid\":\"2d8cca64-5216-4108-8582-3d735b4d6af0\"},{\"content\":{\"connectorIds\":[\"RConn1\"],\"side\":\"BOTTOM\"},\"type\":\"ConnectorPlacement.EquallySpacedRectSide\",\"uuid\":\"da22ed5b-3a7b-44e1-acef-3ebda742cad5\"}]},\"type\":\"ConnectorPlacement.EquallySpacedConnector\",\"uuid\":\"49f96526-0040-486f-9e93-d2a8b3aa1224\"}],\"packageUris\":[\"http://schema.mathworks.com/mf0/Connector/R2020b\"],\"version\":\"1.0\"}"
  Subsystem37 : Subsystem
      settings: PortSchema="{\"entries\":[{\"content\":{\"sides\":[{\"content\":{\"connectorIds\":[\"LConn1\",\"LConn2\"]},\"type\":\"ConnectorPlacement.EquallySpacedRectSide\",\"uuid\":\"15b6a701-c482-4ab4-b894-e969b74b8fe7\"},{\"content\":{\"side\":\"RIGHT\"},\"type\":\"ConnectorPlacement.EquallySpacedRectSide\",\"uuid\":\"d0e695dd-06b6-4831-9b12-69abc92aa4b4\"},{\"content\":{\"connectorIds\":[\"LConn3\"],\"side\":\"TOP\"},\"type\":\"ConnectorPlacement.EquallySpacedRectSide\",\"uuid\":\"2d8cca64-5216-4108-8582-3d735b4d6af0\"},{\"content\":{\"connectorIds\":[\"RConn1\"],\"side\":\"BOTTOM\"},\"type\":\"ConnectorPlacement.EquallySpacedRectSide\",\"uuid\":\"da22ed5b-3a7b-44e1-acef-3ebda742cad5\"}]},\"type\":\"ConnectorPlacement.EquallySpacedConnector\",\"uuid\":\"49f96526-0040-486f-9e93-d2a8b3aa1224\"}],\"packageUris\":[\"http://schema.mathworks.com/mf0/Connector/R2020b\"],\"version\":\"1.0\"}"
  Subsystem38 : Subsystem
      settings: PortSchema="{\"entries\":[{\"content\":{\"sides\":[{\"content\":{\"connectorIds\":[\"LConn1\",\"LConn2\"]},\"type\":\"ConnectorPlacement.EquallySpacedRectSide\",\"uuid\":\"15b6a701-c482-4ab4-b894-e969b74b8fe7\"},{\"content\":{\"side\":\"RIGHT\"},\"type\":\"ConnectorPlacement.EquallySpacedRectSide\",\"uuid\":\"d0e695dd-06b6-4831-9b12-69abc92aa4b4\"},{\"content\":{\"connectorIds\":[\"LConn3\"],\"side\":\"TOP\"},\"type\":\"ConnectorPlacement.EquallySpacedRectSide\",\"uuid\":\"2d8cca64-5216-4108-8582-3d735b4d6af0\"},{\"content\":{\"connectorIds\":[\"RConn1\"],\"side\":\"BOTTOM\"},\"type\":\"ConnectorPlacement.EquallySpacedRectSide\",\"uuid\":\"da22ed5b-3a7b-44e1-acef-3ebda742cad5\"}]},\"type\":\"ConnectorPlacement.EquallySpacedConnector\",\"uuid\":\"49f96526-0040-486f-9e93-d2a8b3aa1224\"}],\"packageUris\":[\"http://schema.mathworks.com/mf0/Connector/R2020b\"],\"version\":\"1.0\"}"
  Subsystem39 : Subsystem
      settings: PortSchema="{\"entries\":[{\"content\":{\"sides\":[{\"content\":{\"connectorIds\":[\"LConn1\",\"LConn2\"]},\"type\":\"ConnectorPlacement.EquallySpacedRectSide\",\"uuid\":\"15b6a701-c482-4ab4-b894-e969b74b8fe7\"},{\"content\":{\"side\":\"RIGHT\"},\"type\":\"ConnectorPlacement.EquallySpacedRectSide\",\"uuid\":\"d0e695dd-06b6-4831-9b12-69abc92aa4b4\"},{\"content\":{\"connectorIds\":[\"LConn3\"],\"side\":\"TOP\"},\"type\":\"ConnectorPlacement.EquallySpacedRectSide\",\"uuid\":\"2d8cca64-5216-4108-8582-3d735b4d6af0\"},{\"content\":{\"connectorIds\":[\"RConn1\"],\"side\":\"BOTTOM\"},\"type\":\"ConnectorPlacement.EquallySpacedRectSide\",\"uuid\":\"da22ed5b-3a7b-44e1-acef-3ebda742cad5\"}]},\"type\":\"ConnectorPlacement.EquallySpacedConnector\",\"uuid\":\"49f96526-0040-486f-9e93-d2a8b3aa1224\"}],\"packageUris\":[\"http://schema.mathworks.com/mf0/Connector/R2020b\"],\"version\":\"1.0\"}"
  Subsystem4 : Subsystem
      settings: PortSchema="{\"entries\":[{\"content\":{\"sides\":[{\"content\":{\"connectorIds\":[\"LConn1\",\"LConn2\"]},\"type\":\"ConnectorPlacement.EquallySpacedRectSide\",\"uuid\":\"15b6a701-c482-4ab4-b894-e969b74b8fe7\"},{\"content\":{\"side\":\"RIGHT\"},\"type\":\"ConnectorPlacement.EquallySpacedRectSide\",\"uuid\":\"d0e695dd-06b6-4831-9b12-69abc92aa4b4\"},{\"content\":{\"connectorIds\":[\"LConn3\"],\"side\":\"TOP\"},\"type\":\"ConnectorPlacement.EquallySpacedRectSide\",\"uuid\":\"2d8cca64-5216-4108-8582-3d735b4d6af0\"},{\"content\":{\"connectorIds\":[\"RConn1\"],\"side\":\"BOTTOM\"},\"type\":\"ConnectorPlacement.EquallySpacedRectSide\",\"uuid\":\"da22ed5b-3a7b-44e1-acef-3ebda742cad5\"}]},\"type\":\"ConnectorPlacement.EquallySpacedConnector\",\"uuid\":\"49f96526-0040-486f-9e93-d2a8b3aa1224\"}],\"packageUris\":[\"http://schema.mathworks.com/mf0/Connector/R2020b\"],\"version\":\"1.0\"}"
  Subsystem40 : Subsystem
      settings: PortSchema="{\"entries\":[{\"content\":{\"sides\":[{\"content\":{\"connectorIds\":[\"LConn1\",\"LConn2\"]},\"type\":\"ConnectorPlacement.EquallySpacedRectSide\",\"uuid\":\"15b6a701-c482-4ab4-b894-e969b74b8fe7\"},{\"content\":{\"side\":\"RIGHT\"},\"type\":\"ConnectorPlacement.EquallySpacedRectSide\",\"uuid\":\"d0e695dd-06b6-4831-9b12-69abc92aa4b4\"},{\"content\":{\"connectorIds\":[\"LConn3\"],\"side\":\"TOP\"},\"type\":\"ConnectorPlacement.EquallySpacedRectSide\",\"uuid\":\"2d8cca64-5216-4108-8582-3d735b4d6af0\"},{\"content\":{\"connectorIds\":[\"RConn1\"],\"side\":\"BOTTOM\"},\"type\":\"ConnectorPlacement.EquallySpacedRectSide\",\"uuid\":\"da22ed5b-3a7b-44e1-acef-3ebda742cad5\"}]},\"type\":\"ConnectorPlacement.EquallySpacedConnector\",\"uuid\":\"49f96526-0040-486f-9e93-d2a8b3aa1224\"}],\"packageUris\":[\"http://schema.mathworks.com/mf0/Connector/R2020b\"],\"version\":\"1.0\"}"
  Subsystem41 : Subsystem
      settings: PortSchema="{\"entries\":[{\"content\":{\"sides\":[{\"content\":{\"connectorIds\":[\"LConn1\",\"LConn2\"]},\"type\":\"ConnectorPlacement.EquallySpacedRectSide\",\"uuid\":\"15b6a701-c482-4ab4-b894-e969b74b8fe7\"},{\"content\":{\"side\":\"RIGHT\"},\"type\":\"ConnectorPlacement.EquallySpacedRectSide\",\"uuid\":\"d0e695dd-06b6-4831-9b12-69abc92aa4b4\"},{\"content\":{\"connectorIds\":[\"LConn3\"],\"side\":\"TOP\"},\"type\":\"ConnectorPlacement.EquallySpacedRectSide\",\"uuid\":\"2d8cca64-5216-4108-8582-3d735b4d6af0\"},{\"content\":{\"connectorIds\":[\"RConn1\"],\"side\":\"BOTTOM\"},\"type\":\"ConnectorPlacement.EquallySpacedRectSide\",\"uuid\":\"da22ed5b-3a7b-44e1-acef-3ebda742cad5\"}]},\"type\":\"ConnectorPlacement.EquallySpacedConnector\",\"uuid\":\"49f96526-0040-486f-9e93-d2a8b3aa1224\"}],\"packageUris\":[\"http://schema.mathworks.com/mf0/Connector/R2020b\"],\"version\":\"1.0\"}"
  Subsystem42 : Subsystem
      settings: PortSchema="{\"entries\":[{\"content\":{\"sides\":[{\"content\":{\"connectorIds\":[\"LConn1\",\"LConn2\"]},\"type\":\"ConnectorPlacement.EquallySpacedRectSide\",\"uuid\":\"15b6a701-c482-4ab4-b894-e969b74b8fe7\"},{\"content\":{\"side\":\"RIGHT\"},\"type\":\"ConnectorPlacement.EquallySpacedRectSide\",\"uuid\":\"d0e695dd-06b6-4831-9b12-69abc92aa4b4\"},{\"content\":{\"connectorIds\":[\"LConn3\"],\"side\":\"TOP\"},\"type\":\"ConnectorPlacement.EquallySpacedRectSide\",\"uuid\":\"2d8cca64-5216-4108-8582-3d735b4d6af0\"},{\"content\":{\"connectorIds\":[\"RConn1\"],\"side\":\"BOTTOM\"},\"type\":\"ConnectorPlacement.EquallySpacedRectSide\",\"uuid\":\"da22ed5b-3a7b-44e1-acef-3ebda742cad5\"}]},\"type\":\"ConnectorPlacement.EquallySpacedConnector\",\"uuid\":\"49f96526-0040-486f-9e93-d2a8b3aa1224\"}],\"packageUris\":[\"http://schema.mathworks.com/mf0/Connector/R2020b\"],\"version\":\"1.0\"}"
  Subsystem43 : Subsystem
      settings: PortSchema="{\"entries\":[{\"content\":{\"sides\":[{\"content\":{\"connectorIds\":[\"LConn1\",\"LConn2\"]},\"type\":\"ConnectorPlacement.EquallySpacedRectSide\",\"uuid\":\"15b6a701-c482-4ab4-b894-e969b74b8fe7\"},{\"content\":{\"side\":\"RIGHT\"},\"type\":\"ConnectorPlacement.EquallySpacedRectSide\",\"uuid\":\"d0e695dd-06b6-4831-9b12-69abc92aa4b4\"},{\"content\":{\"connectorIds\":[\"LConn3\"],\"side\":\"TOP\"},\"type\":\"ConnectorPlacement.EquallySpacedRectSide\",\"uuid\":\"2d8cca64-5216-4108-8582-3d735b4d6af0\"},{\"content\":{\"connectorIds\":[\"RConn1\"],\"side\":\"BOTTOM\"},\"type\":\"ConnectorPlacement.EquallySpacedRectSide\",\"uuid\":\"da22ed5b-3a7b-44e1-acef-3ebda742cad5\"}]},\"type\":\"ConnectorPlacement.EquallySpacedConnector\",\"uuid\":\"49f96526-0040-486f-9e93-d2a8b3aa1224\"}],\"packageUris\":[\"http://schema.mathworks.com/mf0/Connector/R2020b\"],\"version\":\"1.0\"}"
  Subsystem44 : Subsystem
      settings: PortSchema="{\"entries\":[{\"content\":{\"sides\":[{\"content\":{\"connectorIds\":[\"LConn1\",\"LConn2\"]},\"type\":\"ConnectorPlacement.EquallySpacedRectSide\",\"uuid\":\"15b6a701-c482-4ab4-b894-e969b74b8fe7\"},{\"content\":{\"side\":\"RIGHT\"},\"type\":\"ConnectorPlacement.EquallySpacedRectSide\",\"uuid\":\"d0e695dd-06b6-4831-9b12-69abc92aa4b4\"},{\"content\":{\"connectorIds\":[\"LConn3\"],\"side\":\"TOP\"},\"type\":\"ConnectorPlacement.EquallySpacedRectSide\",\"uuid\":\"2d8cca64-5216-4108-8582-3d735b4d6af0\"},{\"content\":{\"connectorIds\":[\"RConn1\"],\"side\":\"BOTTOM\"},\"type\":\"ConnectorPlacement.EquallySpacedRectSide\",\"uuid\":\"da22ed5b-3a7b-44e1-acef-3ebda742cad5\"}]},\"type\":\"ConnectorPlacement.EquallySpacedConnector\",\"uuid\":\"49f96526-0040-486f-9e93-d2a8b3aa1224\"}],\"packageUris\":[\"http://schema.mathworks.com/mf0/Connector/R2020b\"],\"version\":\"1.0\"}"
  Subsystem45 : Subsystem
      settings: PortSchema="{\"entries\":[{\"content\":{\"sides\":[{\"content\":{\"connectorIds\":[\"LConn1\",\"LConn2\"]},\"type\":\"ConnectorPlacement.EquallySpacedRectSide\",\"uuid\":\"15b6a701-c482-4ab4-b894-e969b74b8fe7\"},{\"content\":{\"side\":\"RIGHT\"},\"type\":\"ConnectorPlacement.EquallySpacedRectSide\",\"uuid\":\"d0e695dd-06b6-4831-9b12-69abc92aa4b4\"},{\"content\":{\"connectorIds\":[\"LConn3\"],\"side\":\"TOP\"},\"type\":\"ConnectorPlacement.EquallySpacedRectSide\",\"uuid\":\"2d8cca64-5216-4108-8582-3d735b4d6af0\"},{\"content\":{\"connectorIds\":[\"RConn1\"],\"side\":\"BOTTOM\"},\"type\":\"ConnectorPlacement.EquallySpacedRectSide\",\"uuid\":\"da22ed5b-3a7b-44e1-acef-3ebda742cad5\"}]},\"type\":\"ConnectorPlacement.EquallySpacedConnector\",\"uuid\":\"49f96526-0040-486f-9e93-d2a8b3aa1224\"}],\"packageUris\":[\"http://schema.mathworks.com/mf0/Connector/R2020b\"],\"version\":\"1.0\"}"
  Subsystem46 : Subsystem
      settings: PortSchema="{\"entries\":[{\"content\":{\"sides\":[{\"content\":{\"connectorIds\":[\"LConn1\",\"LConn2\"]},\"type\":\"ConnectorPlacement.EquallySpacedRectSide\",\"uuid\":\"15b6a701-c482-4ab4-b894-e969b74b8fe7\"},{\"content\":{\"side\":\"RIGHT\"},\"type\":\"ConnectorPlacement.EquallySpacedRectSide\",\"uuid\":\"d0e695dd-06b6-4831-9b12-69abc92aa4b4\"},{\"content\":{\"connectorIds\":[\"LConn3\"],\"side\":\"TOP\"},\"type\":\"ConnectorPlacement.EquallySpacedRectSide\",\"uuid\":\"2d8cca64-5216-4108-8582-3d735b4d6af0\"},{\"content\":{\"connectorIds\":[\"RConn1\"],\"side\":\"BOTTOM\"},\"type\":\"ConnectorPlacement.EquallySpacedRectSide\",\"uuid\":\"da22ed5b-3a7b-44e1-acef-3ebda742cad5\"}]},\"type\":\"ConnectorPlacement.EquallySpacedConnector\",\"uuid\":\"49f96526-0040-486f-9e93-d2a8b3aa1224\"}],\"packageUris\":[\"http://schema.mathworks.com/mf0/Connector/R2020b\"],\"version\":\"1.0\"}"
  Subsystem47 : Subsystem
      settings: PortSchema="{\"entries\":[{\"content\":{\"sides\":[{\"content\":{\"connectorIds\":[\"LConn1\",\"LConn2\"]},\"type\":\"ConnectorPlacement.EquallySpacedRectSide\",\"uuid\":\"15b6a701-c482-4ab4-b894-e969b74b8fe7\"},{\"content\":{\"side\":\"RIGHT\"},\"type\":\"ConnectorPlacement.EquallySpacedRectSide\",\"uuid\":\"d0e695dd-06b6-4831-9b12-69abc92aa4b4\"},{\"content\":{\"connectorIds\":[\"LConn3\"],\"side\":\"TOP\"},\"type\":\"ConnectorPlacement.EquallySpacedRectSide\",\"uuid\":\"2d8cca64-5216-4108-8582-3d735b4d6af0\"},{\"content\":{\"connectorIds\":[\"RConn1\"],\"side\":\"BOTTOM\"},\"type\":\"ConnectorPlacement.EquallySpacedRectSide\",\"uuid\":\"da22ed5b-3a7b-44e1-acef-3ebda742cad5\"}]},\"type\":\"ConnectorPlacement.EquallySpacedConnector\",\"uuid\":\"49f96526-0040-486f-9e93-d2a8b3aa1224\"}],\"packageUris\":[\"http://schema.mathworks.com/mf0/Connector/R2020b\"],\"version\":\"1.0\"}"
  Subsystem48 : Subsystem
      settings: PortSchema="{\"entries\":[{\"content\":{\"sides\":[{\"content\":{\"connectorIds\":[\"LConn1\",\"LConn2\"]},\"type\":\"ConnectorPlacement.EquallySpacedRectSide\",\"uuid\":\"15b6a701-c482-4ab4-b894-e969b74b8fe7\"},{\"content\":{\"side\":\"RIGHT\"},\"type\":\"ConnectorPlacement.EquallySpacedRectSide\",\"uuid\":\"d0e695dd-06b6-4831-9b12-69abc92aa4b4\"},{\"content\":{\"connectorIds\":[\"LConn3\"],\"side\":\"TOP\"},\"type\":\"ConnectorPlacement.EquallySpacedRectSide\",\"uuid\":\"2d8cca64-5216-4108-8582-3d735b4d6af0\"},{\"content\":{\"connectorIds\":[\"RConn1\"],\"side\":\"BOTTOM\"},\"type\":\"ConnectorPlacement.EquallySpacedRectSide\",\"uuid\":\"da22ed5b-3a7b-44e1-acef-3ebda742cad5\"}]},\"type\":\"ConnectorPlacement.EquallySpacedConnector\",\"uuid\":\"49f96526-0040-486f-9e93-d2a8b3aa1224\"}],\"packageUris\":[\"http://schema.mathworks.com/mf0/Connector/R2020b\"],\"version\":\"1.0\"}"
  Subsystem5 : Subsystem
      settings: PortSchema="{\"entries\":[{\"content\":{\"sides\":[{\"content\":{\"connectorIds\":[\"LConn1\",\"LConn2\"]},\"type\":\"ConnectorPlacement.EquallySpacedRectSide\",\"uuid\":\"15b6a701-c482-4ab4-b894-e969b74b8fe7\"},{\"content\":{\"side\":\"RIGHT\"},\"type\":\"ConnectorPlacement.EquallySpacedRectSide\",\"uuid\":\"d0e695dd-06b6-4831-9b12-69abc92aa4b4\"},{\"content\":{\"connectorIds\":[\"LConn3\"],\"side\":\"TOP\"},\"type\":\"ConnectorPlacement.EquallySpacedRectSide\",\"uuid\":\"2d8cca64-5216-4108-8582-3d735b4d6af0\"},{\"content\":{\"connectorIds\":[\"RConn1\"],\"side\":\"BOTTOM\"},\"type\":\"ConnectorPlacement.EquallySpacedRectSide\",\"uuid\":\"da22ed5b-3a7b-44e1-acef-3ebda742cad5\"}]},\"type\":\"ConnectorPlacement.EquallySpacedConnector\",\"uuid\":\"49f96526-0040-486f-9e93-d2a8b3aa1224\"}],\"packageUris\":[\"http://schema.mathworks.com/mf0/Connector/R2020b\"],\"version\":\"1.0\"}"
  Subsystem6 : Subsystem
      settings: PortSchema="{\"entries\":[{\"content\":{\"sides\":[{\"content\":{\"connectorIds\":[\"LConn1\",\"LConn2\"]},\"type\":\"ConnectorPlacement.EquallySpacedRectSide\",\"uuid\":\"15b6a701-c482-4ab4-b894-e969b74b8fe7\"},{\"content\":{\"side\":\"RIGHT\"},\"type\":\"ConnectorPlacement.EquallySpacedRectSide\",\"uuid\":\"d0e695dd-06b6-4831-9b12-69abc92aa4b4\"},{\"content\":{\"connectorIds\":[\"LConn3\"],\"side\":\"TOP\"},\"type\":\"ConnectorPlacement.EquallySpacedRectSide\",\"uuid\":\"2d8cca64-5216-4108-8582-3d735b4d6af0\"},{\"content\":{\"connectorIds\":[\"RConn1\"],\"side\":\"BOTTOM\"},\"type\":\"ConnectorPlacement.EquallySpacedRectSide\",\"uuid\":\"da22ed5b-3a7b-44e1-acef-3ebda742cad5\"}]},\"type\":\"ConnectorPlacement.EquallySpacedConnector\",\"uuid\":\"49f96526-0040-486f-9e93-d2a8b3aa1224\"}],\"packageUris\":[\"http://schema.mathworks.com/mf0/Connector/R2020b\"],\"version\":\"1.0\"}"
  Subsystem7 : Subsystem
      settings: PortSchema="{\"entries\":[{\"content\":{\"sides\":[{\"content\":{\"connectorIds\":[\"LConn1\",\"LConn2\"]},\"type\":\"ConnectorPlacement.EquallySpacedRectSide\",\"uuid\":\"15b6a701-c482-4ab4-b894-e969b74b8fe7\"},{\"content\":{\"side\":\"RIGHT\"},\"type\":\"ConnectorPlacement.EquallySpacedRectSide\",\"uuid\":\"d0e695dd-06b6-4831-9b12-69abc92aa4b4\"},{\"content\":{\"connectorIds\":[\"LConn3\"],\"side\":\"TOP\"},\"type\":\"ConnectorPlacement.EquallySpacedRectSide\",\"uuid\":\"2d8cca64-5216-4108-8582-3d735b4d6af0\"},{\"content\":{\"connectorIds\":[\"RConn1\"],\"side\":\"BOTTOM\"},\"type\":\"ConnectorPlacement.EquallySpacedRectSide\",\"uuid\":\"da22ed5b-3a7b-44e1-acef-3ebda742cad5\"}]},\"type\":\"ConnectorPlacement.EquallySpacedConnector\",\"uuid\":\"49f96526-0040-486f-9e93-d2a8b3aa1224\"}],\"packageUris\":[\"http://schema.mathworks.com/mf0/Connector/R2020b\"],\"version\":\"1.0\"}"
  Subsystem8 : Subsystem
      settings: PortSchema="{\"entries\":[{\"content\":{\"sides\":[{\"content\":{\"connectorIds\":[\"LConn1\",\"LConn2\"]},\"type\":\"ConnectorPlacement.EquallySpacedRectSide\",\"uuid\":\"15b6a701-c482-4ab4-b894-e969b74b8fe7\"},{\"content\":{\"side\":\"RIGHT\"},\"type\":\"ConnectorPlacement.EquallySpacedRectSide\",\"uuid\":\"d0e695dd-06b6-4831-9b12-69abc92aa4b4\"},{\"content\":{\"connectorIds\":[\"LConn3\"],\"side\":\"TOP\"},\"type\":\"ConnectorPlacement.EquallySpacedRectSide\",\"uuid\":\"2d8cca64-5216-4108-8582-3d735b4d6af0\"},{\"content\":{\"connectorIds\":[\"RConn1\"],\"side\":\"BOTTOM\"},\"type\":\"ConnectorPlacement.EquallySpacedRectSide\",\"uuid\":\"da22ed5b-3a7b-44e1-acef-3ebda742cad5\"}]},\"type\":\"ConnectorPlacement.EquallySpacedConnector\",\"uuid\":\"49f96526-0040-486f-9e93-d2a8b3aa1224\"}],\"packageUris\":[\"http://schema.mathworks.com/mf0/Connector/R2020b\"],\"version\":\"1.0\"}"
  Subsystem9 : Subsystem
      settings: PortSchema="{\"entries\":[{\"content\":{\"sides\":[{\"content\":{\"connectorIds\":[\"LConn1\",\"LConn2\"]},\"type\":\"ConnectorPlacement.EquallySpacedRectSide\",\"uuid\":\"15b6a701-c482-4ab4-b894-e969b74b8fe7\"},{\"content\":{\"side\":\"RIGHT\"},\"type\":\"ConnectorPlacement.EquallySpacedRectSide\",\"uuid\":\"d0e695dd-06b6-4831-9b12-69abc92aa4b4\"},{\"content\":{\"connectorIds\":[\"LConn3\"],\"side\":\"TOP\"},\"type\":\"ConnectorPlacement.EquallySpacedRectSide\",\"uuid\":\"2d8cca64-5216-4108-8582-3d735b4d6af0\"},{\"content\":{\"connectorIds\":[\"RConn1\"],\"side\":\"BOTTOM\"},\"type\":\"ConnectorPlacement.EquallySpacedRectSide\",\"uuid\":\"da22ed5b-3a7b-44e1-acef-3ebda742cad5\"}]},\"type\":\"ConnectorPlacement.EquallySpacedConnector\",\"uuid\":\"49f96526-0040-486f-9e93-d2a8b3aa1224\"}],\"packageUris\":[\"http://schema.mathworks.com/mf0/Connector/R2020b\"],\"version\":\"1.0\"}"
  Voltage Source : ee_lib/Sources/Voltage Source  dc_voltage=0 V  ac_voltage=0 V  ac_shift=0 rad  ac_frequency=60 Hz  noise_mode=ee.enum.sources.noise.Disabled  PSD=0 V^2/Hz  sample_time=1e-3 s  repeatability=ee.enum.sources.repeatability.NotRepeatable  user_seed=0  auto_seed=3499211588  i_specify=off  i_priority=None  i=0 A  i_nominal_specify=off  i_nominal_value=1  i_nominal_unit=A  v_specify=off  v_priority=None  v=0 V  v_nominal_specify=off  v_nominal_value=1  v_nominal_unit=V
  wires:
  Sine Wave/1 -> MATLAB Function/2(i_ac_ref)
  Constant1/1 -> Simulink-PS Converter1/1
  Constant2/1 -> Simulink-PS Converter2/1
  Constant3/1 -> Simulink-PS Converter3/1
  Constant4/1 -> Simulink-PS Converter4/1
  Constant5/1 -> Simulink-PS Converter5/1
  Constant6/1 -> Simulink-PS Converter6/1
  Constant7/1 -> Simulink-PS Converter7/1
  Constant8/1 -> Simulink-PS Converter8/1
  Constant9/1 -> Simulink-PS Converter9/1
  Constant10/1 -> Simulink-PS Converter10/1
  Constant11/1 -> Simulink-PS Converter11/1
  Constant12/1 -> Simulink-PS Converter12/1
  Constant13/1 -> Simulink-PS Converter13/1
  Constant14/1 -> Simulink-PS Converter14/1
  Constant15/1 -> Simulink-PS Converter15/1
  Constant16/1 -> Simulink-PS Converter16/1
  Constant17/1 -> Simulink-PS Converter17/1
  Constant18/1 -> Simulink-PS Converter18/1
  Constant19/1 -> Simulink-PS Converter19/1
  Constant20/1 -> Simulink-PS Converter20/1
  Constant21/1 -> Simulink-PS Converter21/1
  Constant22/1 -> Simulink-PS Converter22/1
  Constant23/1 -> Simulink-PS Converter23/1
  Constant24/1 -> Simulink-PS Converter24/1
  Constant27/1 -> Simulink-PS Converter27/1
  Constant32/1 -> Simulink-PS Converter32/1
  Constant34/1 -> Simulink-PS Converter34/1
  Constant35/1 -> Simulink-PS Converter35/1
  Constant28/1 -> Simulink-PS Converter28/1
  Constant33/1 -> Simulink-PS Converter33/1
  Constant25/1 -> Simulink-PS Converter25/1
  Constant31/1 -> Simulink-PS Converter31/1
  Constant26/1 -> Simulink-PS Converter26/1
  Constant30/1 -> Simulink-PS Converter30/1
  Constant29/1 -> Simulink-PS Converter29/1
  Constant36/1 -> Simulink-PS Converter36/1
  Constant39/1 -> Simulink-PS Converter39/1
  Constant44/1 -> Simulink-PS Converter44/1
  Constant46/1 -> Simulink-PS Converter46/1
  Constant47/1 -> Simulink-PS Converter47/1
  Constant40/1 -> Simulink-PS Converter40/1
  Constant45/1 -> Simulink-PS Converter45/1
  Constant37/1 -> Simulink-PS Converter37/1
  Constant43/1 -> Simulink-PS Converter43/1
  Constant38/1 -> Simulink-PS Converter38/1
  Constant42/1 -> Simulink-PS Converter42/1
  Constant41/1 -> Simulink-PS Converter41/1
  Constant48/1 -> Simulink-PS Converter48/1
  Constant65/1 -> Simulink-PS Converter65/1
  Constant64/1 -> Simulink-PS Converter64/1
  Constant67/1 -> Simulink-PS Converter67/1
  Constant70/1 -> Simulink-PS Converter70/1
  Constant59/1 -> Simulink-PS Converter59/1
  Constant62/1 -> Simulink-PS Converter62/1
  Constant61/1 -> Simulink-PS Converter61/1
  Constant66/1 -> Simulink-PS Converter66/1
  Constant69/1 -> Simulink-PS Converter69/1
  Constant60/1 -> Simulink-PS Converter60/1
  Constant68/1 -> Simulink-PS Converter68/1
  Constant51/1 -> Simulink-PS Converter51/1
  Constant56/1 -> Simulink-PS Converter56/1
  Constant63/1 -> Simulink-PS Converter63/1
  Constant57/1 -> Simulink-PS Converter57/1
  Constant49/1 -> Simulink-PS Converter49/1
  Constant55/1 -> Simulink-PS Converter55/1
  Constant53/1 -> Simulink-PS Converter53/1
  Constant72/1 -> Simulink-PS Converter72/1
  Constant50/1 -> Simulink-PS Converter50/1
  Constant54/1 -> Simulink-PS Converter54/1
  Constant58/1 -> Simulink-PS Converter58/1
  Constant71/1 -> Simulink-PS Converter71/1
  Constant52/1 -> Simulink-PS Converter52/1
  Constant89/1 -> Simulink-PS Converter89/1
  Constant88/1 -> Simulink-PS Converter88/1
  Constant91/1 -> Simulink-PS Converter91/1
  Constant94/1 -> Simulink-PS Converter94/1
  Constant83/1 -> Simulink-PS Converter83/1
  Constant86/1 -> Simulink-PS Converter86/1
  Constant85/1 -> Simulink-PS Converter85/1
  Constant90/1 -> Simulink-PS Converter90/1
  Constant93/1 -> Simulink-PS Converter93/1
  Constant84/1 -> Simulink-PS Converter84/1
  Constant92/1 -> Simulink-PS Converter92/1
  Constant75/1 -> Simulink-PS Converter75/1
  Constant80/1 -> Simulink-PS Converter80/1
  Constant87/1 -> Simulink-PS Converter87/1
  Constant81/1 -> Simulink-PS Converter81/1
  Constant73/1 -> Simulink-PS Converter73/1
  Constant79/1 -> Simulink-PS Converter79/1
  Constant77/1 -> Simulink-PS Converter77/1
  Constant96/1 -> Simulink-PS Converter96/1
  Constant74/1 -> Simulink-PS Converter74/1
  Constant78/1 -> Simulink-PS Converter78/1
  Constant82/1 -> Simulink-PS Converter82/1
  Constant95/1 -> Simulink-PS Converter95/1
  Constant76/1 -> Simulink-PS Converter76/1
  connections:
  Inductor6/RConn1 -- Resistor/LConn1 -- Inductor7/LConn1
  Simulink-PS Converter1/RConn1 -- Subsystem8/LConn1
  Simulink-PS Converter2/RConn1 -- Subsystem8/LConn2
  Subsystem8/LConn3 -- Inductor7/RConn1
  Simulink-PS Converter3/RConn1 -- Subsystem14/LConn1
  Simulink-PS Converter4/RConn1 -- Subsystem14/LConn2
  Subsystem14/LConn3 -- Subsystem8/RConn1
  Simulink-PS Converter5/RConn1 -- Subsystem15/LConn1
  Simulink-PS Converter6/RConn1 -- Subsystem15/LConn2
  Subsystem15/RConn1 -- Inductor6/LConn1
  Simulink-PS Converter7/RConn1 -- Subsystem16/LConn1
  Simulink-PS Converter8/RConn1 -- Subsystem16/LConn2
  Subsystem15/LConn3 -- Subsystem16/RConn1
  Simulink-PS Converter9/RConn1 -- Subsystem20/LConn1
  Simulink-PS Converter12/RConn1 -- Subsystem17/LConn2
  Simulink-PS Converter11/RConn1 -- Subsystem17/LConn1
  Subsystem17/LConn3 -- Subsystem20/RConn1
  Simulink-PS Converter16/RConn1 -- Subsystem19/LConn2
  Subsystem18/LConn3 -- Subsystem19/RConn1
  Simulink-PS Converter13/RConn1 -- Subsystem18/LConn1
  Inductor8/RConn1 -- Inductor9/LConn1
  Simulink-PS Converter15/RConn1 -- Subsystem19/LConn1
  Simulink-PS Converter10/RConn1 -- Subsystem20/LConn2
  Subsystem18/RConn1 -- Inductor8/LConn1
  Subsystem20/LConn3 -- Inductor9/RConn1
  Simulink-PS Converter14/RConn1 -- Subsystem18/LConn2
  Simulink-PS Converter17/RConn1 -- Subsystem24/LConn1
  Simulink-PS Converter20/RConn1 -- Subsystem21/LConn2
  Simulink-PS Converter19/RConn1 -- Subsystem21/LConn1
  Subsystem21/LConn3 -- Subsystem24/RConn1
  Simulink-PS Converter24/RConn1 -- Subsystem23/LConn2
  Subsystem22/LConn3 -- Subsystem23/RConn1
  Simulink-PS Converter21/RConn1 -- Subsystem22/LConn1
  Inductor10/RConn1 -- Resistor1/LConn1 -- Resistor2/LConn1 -- Inductor11/LConn1
  Simulink-PS Converter23/RConn1 -- Subsystem23/LConn1
  Simulink-PS Converter18/RConn1 -- Subsystem24/LConn2
  Subsystem22/RConn1 -- Inductor10/LConn1
  Subsystem24/LConn3 -- Inductor11/RConn1
  Simulink-PS Converter22/RConn1 -- Subsystem22/LConn2
  Resistor/RConn1 -- Resistor2/RConn1 -- Resistor1/RConn1
  Simulink-PS Converter28/RConn1 -- Subsystem2/LConn2
  Simulink-PS Converter26/RConn1 -- Subsystem3/LConn2
  Simulink-PS Converter32/RConn1 -- Subsystem6/LConn2
  Subsystem1/LConn3 -- Subsystem6/RConn1
  Subsystem3/LConn3 -- Subsystem17/RConn1
  Simulink-PS Converter27/RConn1 -- Subsystem2/LConn1
  Subsystem2/LConn3 -- Subsystem3/RConn1
  Simulink-PS Converter25/RConn1 -- Subsystem6/LConn1
  Simulink-PS Converter31/RConn1 -- Subsystem4/LConn1
  Simulink-PS Converter29/RConn1 -- Subsystem5/LConn1
  Simulink-PS Converter35/RConn1 -- Subsystem1/LConn2
  Simulink-PS Converter33/RConn1 -- Subsystem4/LConn2
  Simulink-PS Converter30/RConn1 -- Subsystem5/LConn2
  Subsystem4/LConn3 -- Subsystem5/RConn1
  Simulink-PS Converter34/RConn1 -- Subsystem1/LConn1
  Subsystem6/LConn3 -- Subsystem14/RConn1
  Subsystem5/LConn3 -- Subsystem21/RConn1
  Simulink-PS Converter36/RConn1 -- Subsystem3/LConn1
  Simulink-PS Converter40/RConn1 -- Subsystem9/LConn2
  Simulink-PS Converter38/RConn1 -- Subsystem10/LConn2
  Simulink-PS Converter44/RConn1 -- Subsystem13/LConn2
  Subsystem7/LConn3 -- Subsystem13/RConn1
  Subsystem10/LConn3 -- Subsystem40/RConn1
  Simulink-PS Converter39/RConn1 -- Subsystem9/LConn1
  Subsystem9/LConn3 -- Subsystem10/RConn1
  Simulink-PS Converter37/RConn1 -- Subsystem13/LConn1
  Simulink-PS Converter43/RConn1 -- Subsystem11/LConn1
  Simulink-PS Converter41/RConn1 -- Subsystem12/LConn1
  Simulink-PS Converter47/RConn1 -- Subsystem7/LConn2
  Simulink-PS Converter45/RConn1 -- Subsystem11/LConn2
  Simulink-PS Converter42/RConn1 -- Subsystem12/LConn2
  Subsystem11/LConn3 -- Subsystem12/RConn1
  Simulink-PS Converter46/RConn1 -- Subsystem7/LConn1
  Subsystem13/LConn3 -- Subsystem37/RConn1
  Subsystem12/LConn3 -- Subsystem45/RConn1
  Simulink-PS Converter48/RConn1 -- Subsystem10/LConn1
  Subsystem16/LConn3 -- Subsystem7/RConn1
  Subsystem19/LConn3 -- Subsystem9/RConn1
  Subsystem23/LConn3 -- Subsystem11/RConn1
  Subsystem32/LConn3 -- Subsystem27/RConn1
  Subsystem33/LConn3 -- Subsystem34/RConn1
  Simulink-PS Converter70/RConn1 -- Subsystem32/LConn1
  Simulink-PS Converter59/RConn1 -- Subsystem32/LConn2
  Subsystem28/LConn3 -- Subsystem32/RConn1
  Simulink-PS Converter64/RConn1 -- Subsystem34/LConn2
  Simulink-PS Converter58/RConn1 -- Subsystem35/LConn1
  Subsystem25/LConn3 -- Subsystem35/RConn1
  Simulink-PS Converter52/RConn1 -- Subsystem27/LConn2
  Simulink-PS Converter61/RConn1 -- Subsystem28/LConn2
  Subsystem27/LConn3 -- Subsystem29/RConn1
  Simulink-PS Converter51/RConn1 -- Subsystem27/LConn1
  Simulink-PS Converter69/RConn1 -- Subsystem25/LConn2
  Simulink-PS Converter72/RConn1 -- Subsystem29/LConn1
  Subsystem35/LConn3 -- Subsystem26/RConn1
  Subsystem34/LConn3 -- Subsystem30/RConn1
  Simulink-PS Converter71/RConn1 -- Subsystem26/LConn2
  Simulink-PS Converter49/RConn1 -- Subsystem36/LConn1
  Simulink-PS Converter50/RConn1 -- Subsystem29/LConn2
  Simulink-PS Converter65/RConn1 -- Subsystem33/LConn1
  Subsystem26/LConn3 -- Subsystem36/RConn1
  Simulink-PS Converter68/RConn1 -- Subsystem25/LConn1
  Simulink-PS Converter55/RConn1 -- Subsystem30/LConn1
  Simulink-PS Converter62/RConn1 -- Subsystem34/LConn1
  Simulink-PS Converter53/RConn1 -- Subsystem31/LConn1
  Simulink-PS Converter66/RConn1 -- Subsystem35/LConn2
  Simulink-PS Converter63/RConn1 -- Subsystem26/LConn1
  Simulink-PS Converter67/RConn1 -- Subsystem33/LConn2
  Subsystem30/LConn3 -- Subsystem31/RConn1
  Simulink-PS Converter60/RConn1 -- Subsystem28/LConn1
  Simulink-PS Converter57/RConn1 -- Subsystem30/LConn2
  Simulink-PS Converter56/RConn1 -- Subsystem36/LConn2
  Simulink-PS Converter54/RConn1 -- Subsystem31/LConn2
  Subsystem36/LConn3 -- Subsystem1/RConn1
  Subsystem29/LConn3 -- Subsystem2/RConn1
  Subsystem31/LConn3 -- Subsystem4/RConn1
  Subsystem44/LConn3 -- Subsystem39/RConn1
  Subsystem45/LConn3 -- Subsystem46/RConn1
  Simulink-PS Converter94/RConn1 -- Subsystem44/LConn1
  Simulink-PS Converter83/RConn1 -- Subsystem44/LConn2
  Subsystem40/LConn3 -- Subsystem44/RConn1
  Simulink-PS Converter88/RConn1 -- Subsystem46/LConn2
  Simulink-PS Converter82/RConn1 -- Subsystem47/LConn1
  Subsystem37/LConn3 -- Subsystem47/RConn1
  Simulink-PS Converter76/RConn1 -- Subsystem39/LConn2
  Simulink-PS Converter85/RConn1 -- Subsystem40/LConn2
  Subsystem39/LConn3 -- Subsystem41/RConn1
  Simulink-PS Converter75/RConn1 -- Subsystem39/LConn1
  Simulink-PS Converter93/RConn1 -- Subsystem37/LConn2
  Simulink-PS Converter96/RConn1 -- Subsystem41/LConn1
  Subsystem47/LConn3 -- Subsystem38/RConn1
  Subsystem46/LConn3 -- Subsystem42/RConn1
  Simulink-PS Converter95/RConn1 -- Subsystem38/LConn2
  Simulink-PS Converter73/RConn1 -- Subsystem48/LConn1
  Simulink-PS Converter74/RConn1 -- Subsystem41/LConn2
  Simulink-PS Converter89/RConn1 -- Subsystem45/LConn1
  Subsystem38/LConn3 -- Subsystem48/RConn1
  Simulink-PS Converter92/RConn1 -- Subsystem37/LConn1
  Simulink-PS Converter79/RConn1 -- Subsystem42/LConn1
  Simulink-PS Converter86/RConn1 -- Subsystem46/LConn1
  Simulink-PS Converter77/RConn1 -- Subsystem43/LConn1
  Simulink-PS Converter90/RConn1 -- Subsystem47/LConn2
  Simulink-PS Converter87/RConn1 -- Subsystem38/LConn1
  Simulink-PS Converter91/RConn1 -- Subsystem45/LConn2
  Subsystem42/LConn3 -- Subsystem43/RConn1
  Simulink-PS Converter84/RConn1 -- Subsystem40/LConn1
  Simulink-PS Converter81/RConn1 -- Subsystem42/LConn2
  Simulink-PS Converter80/RConn1 -- Subsystem48/LConn2
  Simulink-PS Converter78/RConn1 -- Subsystem43/LConn2
  Subsystem48/LConn3 -- Voltage Source/LConn1 -- Subsystem43/LConn3 -- Subsystem41/LConn3
  Subsystem28/RConn1 -- Voltage Source/RConn1 -- Subsystem25/RConn1 -- Electrical Reference/LConn1 -- Solver Configuration1/RConn1 -- Subsystem33/RConn1
